simulink model "unballance_pod_trav"  (R2022b)
settings: Solver=VariableStepAuto  StartTime=0.0  StopTime=10.0  RelTol=1e-3
settings Model: Creator=ohadformanair  LastModifiedBy=ohadformanair

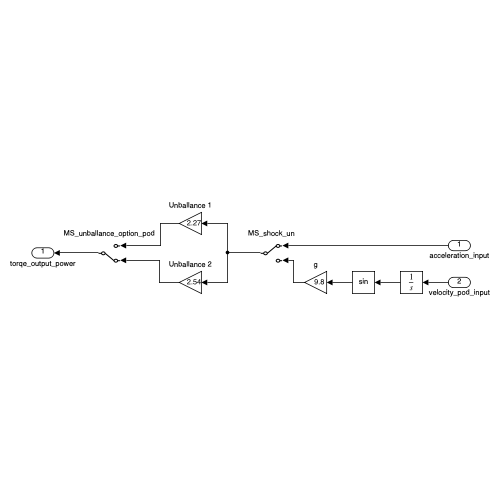
[thumbnail: Simulink's stored preview of the top-level diagram]
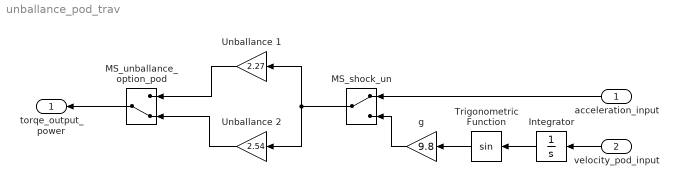
== system unballance_pod_trav ==
  acceleration_input : Inport
  velocity_pod_input : Inport  Port=2
  Integrator : Integrator
  MS_shock_un : ManualSwitch
  MS_unballance_option_pod : ManualSwitch  CurrentSetting=0
  Trigonometric Function : Trigonometry
  Unballance 1 : Gain  Gain=2.27
  Unballance 2 : Gain  Gain=2.54
  g : Gain  Gain=9.8
  torqe_output_power : Outport
  wires:
  MS_unballance_option_pod/1 -> torqe_output_power/1
  Integrator/1 -> Trigonometric Function/1
  Unballance 2/1 -> MS_unballance_option_pod/2
  g/1 -> MS_shock_un/2
  Unballance 1/1 -> MS_unballance_option_pod/1
  Trigonometric Function/1 -> g/1
  velocity_pod_input/1 -> Integrator/1
  MS_shock_un/1 -> Unballance 2/1, Unballance 1/1
  acceleration_input/1 -> MS_shock_un/1
